simulink subsystem "MPC"  (R2025b)
settings: Solver=VariableStepAuto  StartTime=0.0  StopTime=10.0  RelTol=1e-3
values from neighbouring files (symbols this model uses):
  Q = diag([Cost_rb Cost_V Cost_I])    [LQG_Integral.m]
  x0_bar = [E0; P0; T0; zeros(nx+nz-3, 1)]    [LQG_Integral.m]
undefined symbols (not defined in the file or in its folder): DAC_lim_u, DiscIntNeverNeededParam, Discrete, K_r, l, N, nu, nx, q, QN, R_kalman, Time, Ts, U_e_real, x_opt_ref_i
libraries: ctrlSharedLib x1
settings Model: Creator=leeta  LastModifiedBy=leeta

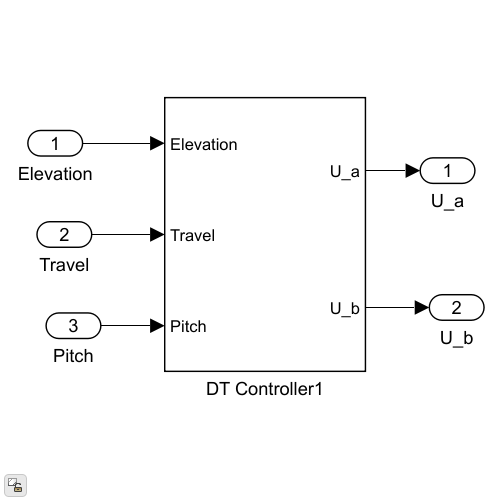
[thumbnail: Simulink's stored preview of the top-level diagram]
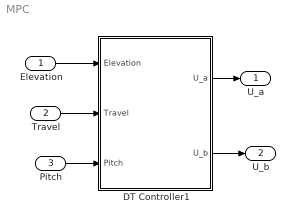
== system MPC ==
  Elevation : Inport
  Travel : Inport  Port=2
  Pitch : Inport  Port=3
  DT Controller1 : Subsystem
  U_a : Outport
  U_b : Outport  Port=2
  wires:
  Travel/1 -> DT Controller1/2(Travel)
  Elevation/1 -> DT Controller1/1(Elevation)
  DT Controller1/2(U_b) -> U_b/1
  Pitch/1 -> DT Controller1/3(Pitch)
  DT Controller1/1(U_a) -> U_a/1

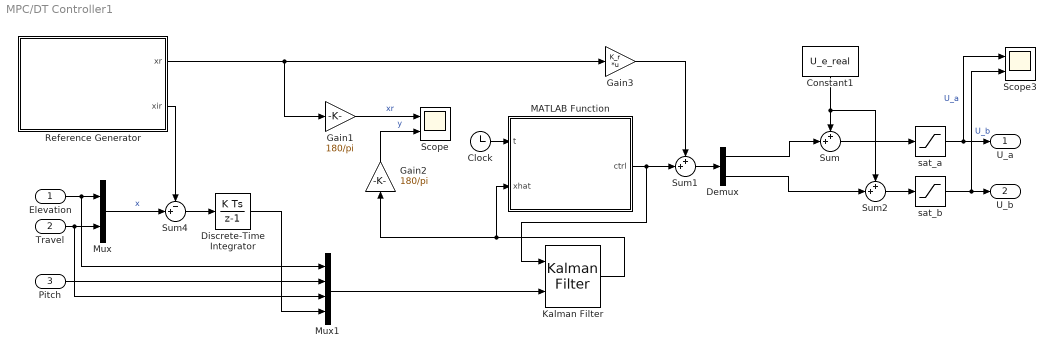
== system MPC/DT Controller1 ==
  Elevation : Inport
  Travel : Inport  Port=2
  Pitch : Inport  Port=3
  Clock : Clock
  Constant1 : Constant  Value=U_e_real
  Demux : Demux  Outputs=2
  Discrete-Time Integrator : DiscreteIntegrator  SampleTime=-1  ICPrevOutput=DiscIntNeverNeededParam  ICPrevScaledInput=DiscIntNeverNeededParam
  Gain1 : Gain  Gain=180/pi
  Gain2 : Gain  Gain=180/pi
  Gain3 : Gain  Gain=K_r  Multiplication=Matrix(K*u)
  Kalman Filter : ctrlSharedLib/Kalman Filter  TimeDomain=Discrete-Time  UseCurrentEstimator=on  ModelSource=LTI State-Space Variable  ModelSourceVariable=sysdt_bar  A=0.95  B=1  C=1  D=0  NumberOfStates=1  NumberOfInputs=1  NumberOfOutputs=1  InitialEstimateSource=Dialog  X0=x0_bar  P0=10  UseK=off  UseGH=off  NumberOfProcessNoiseInputs=1  G=1  TimeInvariantG=on  H=0  TimeInvariantH=on  Q=1  TimeInvariantQ=on  R=R_kalman  TimeInvariantR=on  N=0  TimeInvariantN=on  AddInputPort=on  AddEnablePort=off  OutputEstimatedY=off  OutputP=off  Ts=-1
  MATLAB Function : MATLAB Function  TreatAsAtomicUnit=on
  Mux : Mux  Inputs=2
  Mux1 : Mux
  Reference Generator : Subsystem  Variant=on
  Scope : Scope  NumInputPorts=2
      settings: ActiveDisplayYMinimum=-47.889888660818315  ActiveDisplayYMaximum=249.78511133915242
  Scope3 : Scope  NumInputPorts=2
      settings: ActiveDisplayYMinimum=-6.1994733501463131  ActiveDisplayYMaximum=15.321917902160504  DataLoggingVariableName=ScopeData6
  Sum : Sum  Inputs=++|
  Sum1 : Sum  Inputs=++|
  Sum2 : Sum  Inputs=++|
  Sum4 : Sum  Inputs=-+|
  sat_a : Saturate  UpperLimit=DAC_lim_u  LowerLimit=0
  sat_b : Saturate  UpperLimit=DAC_lim_u  LowerLimit=0
  U_a : Outport
  U_b : Outport  Port=2
  wires:
  Clock/1 -> MATLAB Function/1(t)
  Discrete-Time Integrator/1 -> Mux1/4
  Gain3/1 -> Sum1/1
  Sum1/1 -> Demux/1
  Reference Generator/2(xir) -> Sum4/1
  Reference Generator/1(xr) -> Gain3/1, Gain1/1
  Gain2/1 -> Scope/2  "y"
  Gain1/1 -> Scope/1  "xr"
  Sum4/1 -> Discrete-Time Integrator/1
  Mux1/1 -> Kalman Filter/2
  Pitch/1 -> Mux1/2
  Mux/1 -> Sum4/2  "x"
  Constant1/1 -> Sum/1, Sum2/1
  Sum2/1 -> sat_b/1
  Sum/1 -> sat_a/1
  Demux/2 -> Sum2/2
  Demux/1 -> Sum/2
  MATLAB Function/1(ctrl) -> Sum1/2, Kalman Filter/1
  Kalman Filter/1 -> Gain2/1, MATLAB Function/2(xhat)
  Travel/1 -> Mux/2, Mux1/3
  Elevation/1 -> Mux/1, Mux1/1
  sat_a/1 -> U_a/1, Scope3/1  "U_a"
  sat_b/1 -> U_b/1, Scope3/2  "U_b"

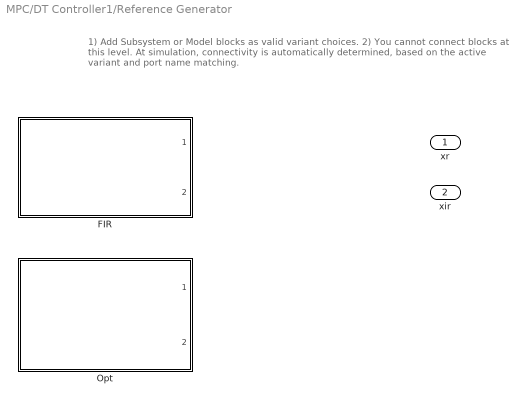
== system MPC/DT Controller1/Reference Generator ==
  note: 1) Add Subsystem or Model blocks as valid variant choices.
      | 2) You cannot connect blocks at this level. At simulation, connectivity is automatically
      | determined, based on the active variant and port name matching.
  FIR : Subsystem  VariantControl=ref_v ==2  ReferencedSubsystem=FIRReferenceGenerator
  Opt : Subsystem  VariantControl=ref_v==1  ReferencedSubsystem=OptimalReferenceGenerator
  xr : Outport
  xir : Outport  Port=2

== matlab function MPC/DT Controller1/MATLAB Function ==
  settings: updateMethod=DISCRETE
  data: t input double size=1; xhat input double size=nx; ctrl output double size=nu; l parameter; u parameter; q parameter; Q parameter; QN parameter; nx parameter; nu parameter; N parameter; x_opt_ref_i parameter; Ts parameter
function ctrl = mpc_step(t, xhat, l, u, q, Q, QN, nx, nu, N, x_opt_ref_i, Ts)

    coder.extrinsic('emosqp')
    
    % Update initial state
    l(1:nx) = -xhat;
    u(1:nx) = -xhat;

    n = round(t/Ts) + 1;

    % if (mod(n,100) == 0) disp(n)

    % Grab the reference from now till the end of horizon (-1 for QN)
    % -> multiply by Q to get the cost
    Qxr = -Q*x_opt_ref_i(:, n:n+N-1);
    Qxrn = -QN*x_opt_ref_i(:, n+N); % For terminal cost

    % Reshape so it's stacked vertically
    Qxr = reshape(Qxr, nx*N, 1);

    q = [Qxrn; Qxr; zeros(N*nu, 1)];

    % Update cost for variable xr
    % q = [repmat(-Q*xr, N, 1); -QN*xr; zeros(N*nu, 1)];

    % Update OSQP problem
    emosqp('update_bounds', l, u);
    emosqp('update_lin_cost', q);

    [x, ~, ~, ~, ~] = emosqp('solve'); 

    ctrl = x((N+1)*nx+1:(N+1)*nx+nu);
    % ctrl(1) = ctrl(1) + U_e;
    % ctrl(2) = ctrl(2) + U_e;
end
